simulink model "Stator_flux_DTC"  (R2018b)
settings: Solver=ode4  StartTime=0.0  StopTime=0.5  FixedStep=1e-5  RelTol=1e-5
libraries: powerlib x6, simulink x1
settings Model: Creator=疯歌小孔丘  LastModifiedBy=疯歌小孔丘

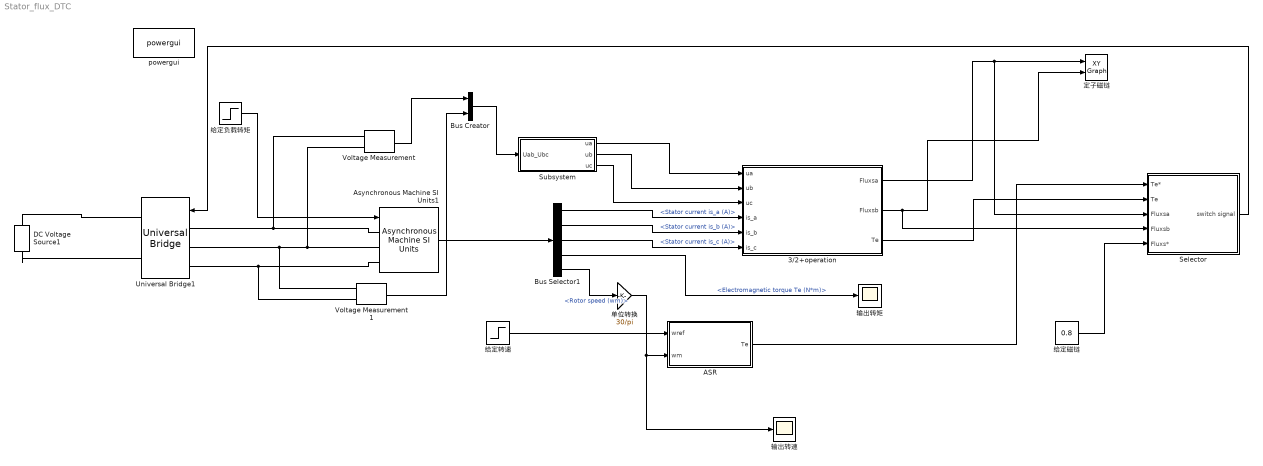
== system Stator_flux_DTC ==
  3/2+operation : Subsystem
  ASR : Subsystem
  Asynchronous Machine SI Units1 : powerlib/Machines/Asynchronous Machine SI Units  RotorType=Squirrel-cage  PresetModel="17:  20 HP (15KW)   400 V 50Hz 1460 RPM"  MechanicalLoad=Torque Tm  ShowDetailedParameters=on  ReferenceFrame=Stationary  Units=SI  MeasurementBus=off  NominalParameters=[1.5e+04 400 50]  Stator=[0.2147 0.000991]  Rotor=[0.2205 0.000991]  Cage1=[ 0.022 0.226/377]  Cage2=[ 0.022 0.226/377]  Lm=0.06419  Mechanical=[0.102 0.009541 2]  PolePairs=2  InitialConditions="[ 1,0   0,0,0   0,0,0 ]"  SimulateSaturation=off  Saturation=[9.9249,19.6672,38.0377,51.3988,69.2824,105.1337,152.5532,214.2421,303.1917;230, 322, 414, 460, 506, 552, 598, 644, 690]  LoadFlowParameters=0  TsPowergui=0  TsBlock=-1  IterativeModel=Forward Euler  IterativeDiscreteModel=Trapezoidal non iterative  Pmec=0
  Bus Creator : BusCreator  Inputs=2
  Bus Selector1 : BusSelector  OutputSignals=Stator measurements.Stator current is_a (A),Stator measurements.Stator current is_b (A),Stator measurements.Stator current is_c (A),Mechanical.Electromagnetic torque Te (N*m),Mechanical.Rotor speed (wm)
  DC Voltage Source1 : powerlib/Electrical Sources/DC Voltage Source  Amplitude=400  Measurements=None
  Selector : Subsystem
  Subsystem : Subsystem
  Universal Bridge1 : powerlib/Power Electronics/Universal Bridge  Arms=3  SnubberResistance=1e5  SnubberCapacitance=inf  Device=IGBT / Diodes  Ron=1e-3  Lon=0  ForwardVoltages="[  0  0  ]"  ForwardVoltage=0  GTOparameters=[ 10e-6 , 20e-6 ]  IGBTparameters=[ 1e-6 , 2e-6 ]  Measurements=None  Measurements_2=None  converterType=Rectifier
  Voltage Measurement : powerlib/Measurements/Voltage Measurement  PhasorSimulation=off  OutputType=Complex  PSBequivalent=0
  Voltage Measurement1 : powerlib/Measurements/Voltage Measurement  PhasorSimulation=off  OutputType=Complex  PSBequivalent=0
  powergui : powerlib/powergui  Priority=1  SimulationMode=Continuous  SampleTime=50e-6  frequency=60  Iterations=50  frequencyindice=50  Pbase=100e6  ErrMax=1e-4  UnitsV=kV  UnitsW=MW  buscounter=0  FunctionMessages=off  echomessages=off  EnableUseOfTLC=off  CurrentSourceSwitches=off  DisableSnubberDevices=off  DisableRonSwitches=off  DisableVfSwitches=off  DisplayEquations=off  SolverType=Tustin/Backward Euler (TBE)  Interpol=off  ExternalGateDelay=off  methode=off  Ts=100  x0status=blocks  SPID=on  SwTol=0  HookPort=off  RestoreLinks=warning  ResistiveCurrentMeasurement=off  Frange=[0:2:500]  Ylog=off  Xlog=on  ShowGrid=off  save=off  variable=ZData  structure=0  ZoomFFT=off  StartTime=0.0  cycles=1  DisplayStyle=1  fundamental=60  FreqAxis=off  MaxFrequency=1000  frequencyindicesteady=1  RmsSteady=1  display=off
  单位转换 : Gain  Gain=30/pi
  定子磁链 : simulink/Sinks/XY Graph  xmin=-1  xmax=1  ymin=-1  ymax=1  st=-1
  给定磁链 : Constant  Value=0.8
  给定负载转矩 : Step  Time=0.2  Before=50  After=60  SampleTime=0
  给定转速 : Step  Time=0.1  Before=100  After=120  SampleTime=0
  输出转矩 : Scope
  输出转速 : Scope
  wires:
  给定转速/1 -> ASR/1("wref ")
  Voltage Measurement1/1 -> Bus Creator/2
  ASR/1(Te) -> Selector/1(Te*)
  Voltage Measurement/1 -> Bus Creator/1
  Bus Creator/1 -> Subsystem/1(Uab_Ubc)
  给定磁链/1 -> Selector/5(Fluxs*)
  Subsystem/1(ua) -> 3/2+operation/1("ua ")
  Subsystem/2(ub) -> 3/2+operation/2(ub)
  Subsystem/3(uc) -> 3/2+operation/3(uc)
  Bus Selector1/1 -> 3/2+operation/4("is_a ")  "<Stator current is_a (A)>"
  Bus Selector1/2 -> 3/2+operation/5(is_b)  "<Stator current is_b (A)>"
  Bus Selector1/3 -> 3/2+operation/6(is_c)  "<Stator current is_c (A)>"
  Bus Selector1/4 -> 输出转矩/1  "<Electromagnetic torque Te (N*m)>"
  Selector/1(switch signal) -> Universal Bridge1/1
  给定负载转矩/1 -> Asynchronous Machine SI Units1/1
  Asynchronous Machine SI Units1/1 -> Bus Selector1/1
  3/2+operation/3(Te) -> Selector/2(Te)
  3/2+operation/2(Fluxsb) -> Selector/4(Fluxsb), 定子磁链/2
  3/2+operation/1(Fluxsa) -> Selector/3(Fluxsa), 定子磁链/1
  Bus Selector1/5 -> 单位转换/1  "<Rotor speed (wm)>"
  单位转换/1 -> ASR/2(wm), 输出转速/1
  connections:
  DC Voltage Source1/RConn1 -- Universal Bridge1/RConn1
  DC Voltage Source1/LConn1 -- Universal Bridge1/RConn2
  Universal Bridge1/LConn1 -- Voltage Measurement/LConn1 -- Asynchronous Machine SI Units1/LConn1
  Universal Bridge1/LConn2 -- Voltage Measurement1/LConn1 -- Asynchronous Machine SI Units1/LConn2 -- Voltage Measurement/LConn2
  Universal Bridge1/LConn3 -- Voltage Measurement1/LConn2 -- Asynchronous Machine SI Units1/LConn3

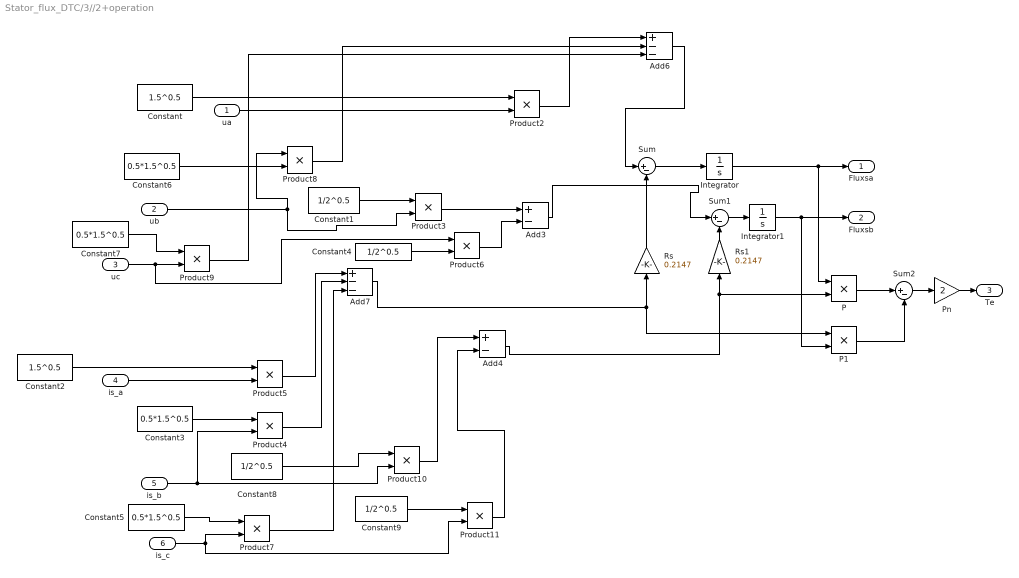
== system Stator_flux_DTC/3//2+operation ==
  "ua " : Inport
  ub : Inport  Port=2
  uc : Inport  Port=3
  "is_a " : Inport  Port=4
  is_b : Inport  Port=5
  is_c : Inport  Port=6
  Add3 : Sum  Inputs=+-
  Add4 : Sum  Inputs=+-
  Add6 : Sum  Inputs=+--
  Add7 : Sum  Inputs=+--
  Constant : Constant  Value=1.5^0.5
  Constant{1,4,8..9} (4 alike) : Constant  Value=1/2^0.5
  Constant2 : Constant  Value=1.5^0.5
  Constant{3,5..7} (4 alike) : Constant  Value=0.5*1.5^0.5
  Integrator : Integrator  InitialCondition=0.001  LimitOutput=on  UpperSaturationLimit=1e6  LowerSaturationLimit=-1e6
  Integrator1 : Integrator  InitialCondition=0.001  LimitOutput=on  UpperSaturationLimit=1e6  LowerSaturationLimit=-1e6
  P : Product  Inputs=**
  P1 : Product  Inputs=**
  Pn : Gain  Gain=2
  Product{2..11} (10 alike) : Product
  Rs : Gain  Gain=0.2147
  Rs1 : Gain  Gain=0.2147
  Sum : Sum  Inputs=|+-
  Sum1 : Sum  Inputs=|+-
  Sum2 : Sum  Inputs=|+-
  Fluxsa : Outport
  Fluxsb : Outport  Port=2
  Te : Outport  Port=3
  wires:
  Constant/1 -> Product2/1
  "ua "/1 -> Product2/2
  ub/1 -> Product3/2, Product8/1
  Constant1/1 -> Product3/1
  Product3/1 -> Add3/1
  Constant6/1 -> Product8/2
  Product2/1 -> Add6/1
  Product8/1 -> Add6/2
  uc/1 -> Product6/1, Product9/2
  Constant7/1 -> Product9/1
  Product9/1 -> Add6/3
  Constant4/1 -> Product6/2
  Product6/1 -> Add3/2
  "is_a "/1 -> Product5/2
  Constant2/1 -> Product5/1
  Product5/1 -> Add7/1
  Constant3/1 -> Product4/1
  is_b/1 -> Product10/2, Product4/2
  Product4/1 -> Add7/2
  Constant5/1 -> Product7/1
  is_c/1 -> Product7/2, Product11/2
  Product7/1 -> Add7/3
  Constant8/1 -> Product10/1
  Product10/1 -> Add4/1
  Constant9/1 -> Product11/1
  Product11/1 -> Add4/2
  Sum/1 -> Integrator/1
  Sum2/1 -> Pn/1
  Sum1/1 -> Integrator1/1
  Integrator/1 -> P/1, Fluxsa/1
  Rs1/1 -> Sum1/2
  Integrator1/1 -> P1/2, Fluxsb/1
  Pn/1 -> Te/1
  Add4/1 -> P/2, Rs1/1
  Add7/1 -> Rs/1, P1/1
  Rs/1 -> Sum/2
  Add3/1 -> Sum1/1
  P1/1 -> Sum2/2
  Add6/1 -> Sum/1
  P/1 -> Sum2/1

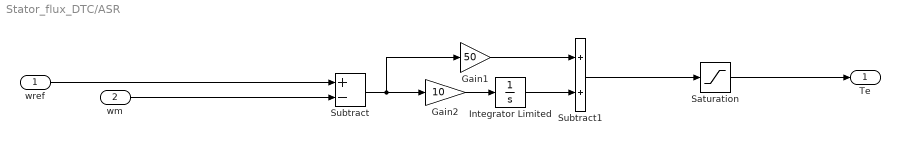
== system Stator_flux_DTC/ASR ==
  "wref " : Inport
  wm : Inport  Port=2
  Gain1 : Gain  Gain=50
  Gain2 : Gain  Gain=10  OutMin=[-200]  OutMax=[200]
  Integrator Limited : Integrator  LimitOutput=on  UpperSaturationLimit=120  LowerSaturationLimit=-120
  Saturation : Saturate  UpperLimit=120  LowerLimit=-120
  Subtract : Sum  Inputs=+-
  Subtract1 : Sum
  Te : Outport
  wires:
  Integrator Limited/1 -> Subtract1/2
  "wref "/1 -> Subtract/1
  Gain1/1 -> Subtract1/1
  Subtract/1 -> Gain1/1, Gain2/1
  Gain2/1 -> Integrator Limited/1
  Subtract1/1 -> Saturation/1
  wm/1 -> Subtract/2
  Saturation/1 -> Te/1

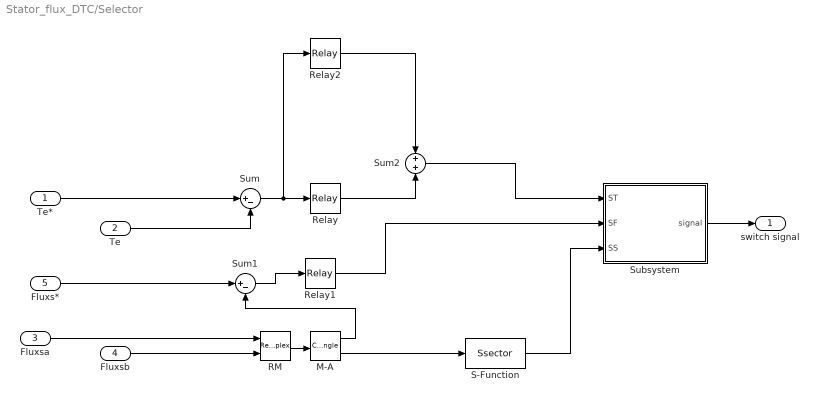
== system Stator_flux_DTC/Selector ==
  Te* : Inport
  Te : Inport  Port=2
  Fluxsa : Inport  Port=3
  Fluxsb : Inport  Port=4
  Fluxs* : Inport  Port=5
  M-A : ComplexToMagnitudeAngle
  RM : RealImagToComplex
  Relay : Relay  OnSwitchValue=0  OffSwitchValue=-1e-9  OnOutputValue=0  OffOutputValue=-1
  Relay1 : Relay  OnSwitchValue=1e-9  OffSwitchValue=-1e-9
  Relay2 : Relay  OnSwitchValue=1e-9  OffSwitchValue=0
  S-Function : S-Function  FunctionName=Ssector  SFunctionDeploymentMode=off  EnableBusSupport=off
  Subsystem : Subsystem
  Sum : Sum  Inputs=|+-
  Sum1 : Sum  Inputs=|+-
  Sum2 : Sum
  switch signal : Outport
  wires:
  Subsystem/1(signal) -> switch signal/1
  Relay1/1 -> Subsystem/2(SF)
  Fluxsb/1 -> RM/2
  Sum1/1 -> Relay1/1
  M-A/1 -> Sum1/2
  Fluxs*/1 -> Sum1/1
  RM/1 -> M-A/1
  Fluxsa/1 -> RM/1
  Sum/1 -> Relay2/1, Relay/1
  Te/1 -> Sum/2
  Te*/1 -> Sum/1
  M-A/2 -> S-Function/1
  S-Function/1 -> Subsystem/3(SS)
  Relay/1 -> Sum2/2
  Relay2/1 -> Sum2/1
  Sum2/1 -> Subsystem/1(ST)

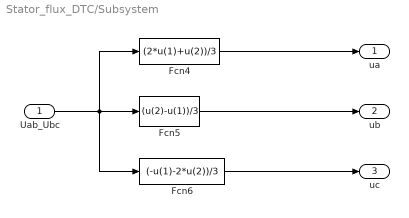
== system Stator_flux_DTC/Subsystem ==
  Uab_Ubc : Inport
  Fcn4 : Fcn  Expr=(2*u(1)+u(2))/3
  Fcn5 : Fcn  Expr=(u(2)-u(1))/3
  Fcn6 : Fcn  Expr=(-u(1)-2*u(2))/3
  ua : Outport
  ub : Outport  Port=2
  uc : Outport  Port=3
  wires:
  Uab_Ubc/1 -> Fcn5/1, Fcn4/1, Fcn6/1
  Fcn4/1 -> ua/1
  Fcn5/1 -> ub/1
  Fcn6/1 -> uc/1

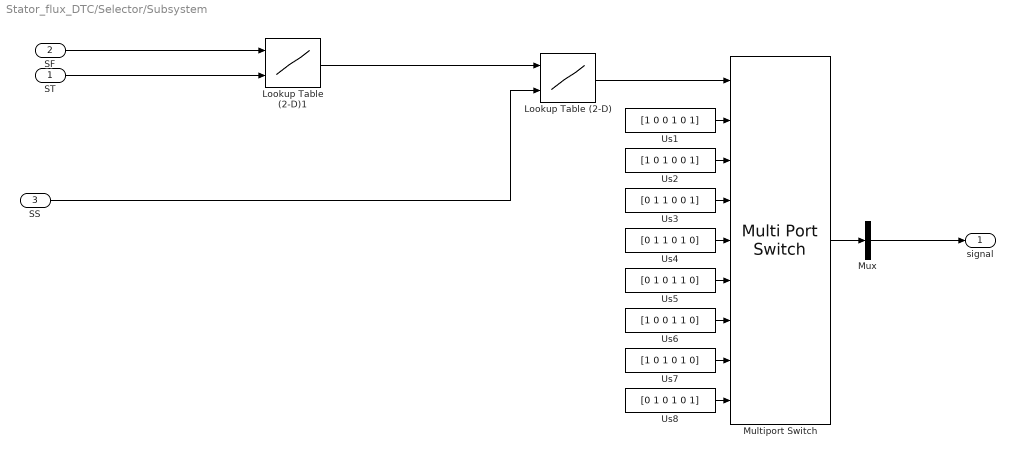
== system Stator_flux_DTC/Selector/Subsystem ==
  ST : Inport
  SF : Inport  Port=2
  SS : Inport  Port=3
  Lookup Table (2-D) : Lookup2D  RowIndex=[1;2;3;4;5;6]  ColumnIndex=[1;2;3;4;5;6]  Table=[ 5 6 1 2 3 4;8 7 8 7 8 7;3 4 5 6 1 2;6 1 2 3 4 5;7 8 7 8 7 8;2 3 4 5 6 1]
  Lookup Table (2-D)1 : Lookup2D  ColumnIndex=[-1 0 1]  Table=[1 2 3; 4 5 6]
  Multiport Switch : MultiPortSwitch  Inputs=8
  Mux : Mux  Inputs=1
  Us1 : Constant  Value=[1 0 0 1 0 1]
  Us2 : Constant  Value=[1 0 1 0 0 1]
  Us3 : Constant  Value=[0 1 1 0 0 1]
  Us4 : Constant  Value=[0 1 1 0 1 0]
  Us5 : Constant  Value=[0 1 0 1 1 0]
  Us6 : Constant  Value=[1 0 0 1 1 0]
  Us7 : Constant  Value=[1 0 1 0 1 0]
  Us8 : Constant  Value=[0 1 0 1 0 1]
  signal : Outport
  wires:
  Mux/1 -> signal/1
  Multiport Switch/1 -> Mux/1
  Us8/1 -> Multiport Switch/9
  Us7/1 -> Multiport Switch/8
  Us6/1 -> Multiport Switch/7
  Us5/1 -> Multiport Switch/6
  Us4/1 -> Multiport Switch/5
  Us3/1 -> Multiport Switch/4
  Us2/1 -> Multiport Switch/3
  Us1/1 -> Multiport Switch/2
  Lookup Table (2-D)/1 -> Multiport Switch/1
  SS/1 -> Lookup Table (2-D)/2
  Lookup Table (2-D)1/1 -> Lookup Table (2-D)/1
  ST/1 -> Lookup Table (2-D)1/2
  SF/1 -> Lookup Table (2-D)1/1
